simulink model "Problem4"  (R2020a)
settings: Solver=VariableStepAuto  StartTime=0.0  StopTime=10.0  FixedStep=1  RelTol=1e-3
settings Model: Creator=Jake  LastModifiedBy=Jake

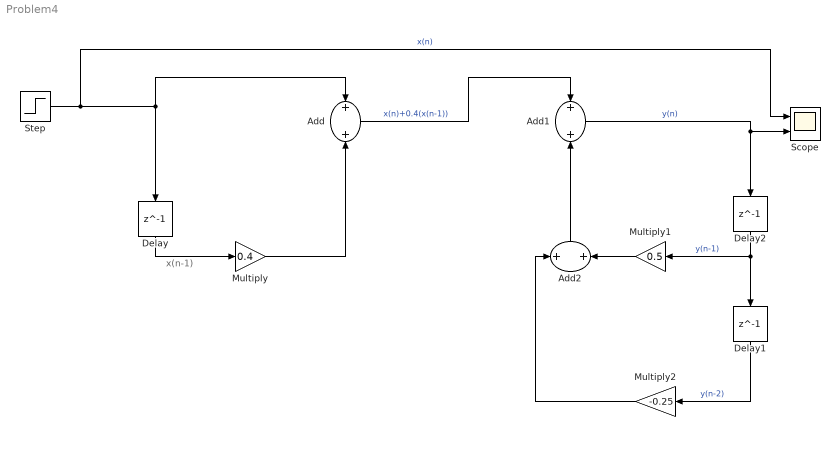
== system Problem4 ==
  note: x(n-1)
  Add : Sum
  Add1 : Sum
  Add2 : Sum
  Delay : Delay  DelayLength=1
  Delay1 : Delay  DelayLength=1
  Delay2 : Delay  DelayLength=1
  Multiply : Gain  Gain=0.4
  Multiply1 : Gain  Gain=0.5
  Multiply2 : Gain  Gain=-0.25
  Scope : Scope  NumInputPorts=2
  Step : Step  After=2  SampleTime=0.01
  wires:
  Step/1 -> Scope/1, Add/1, Delay/1  "x(n)"
  Delay/1 -> Multiply/1
  Multiply/1 -> Add/2
  Add/1 -> Add1/1  "x(n)+0.4(x(n-1))"
  Add1/1 -> Delay2/1, Scope/2  "y(n)"
  Delay2/1 -> Multiply1/1, Delay1/1  "y(n-1)"
  Delay1/1 -> Multiply2/1  "y(n-2)"
  Multiply1/1 -> Add2/2
  Multiply2/1 -> Add2/1
  Add2/1 -> Add1/2
